simulink model "proyectolab"  (R2020a)
settings: Solver=FixedStepAuto  StartTime=0.0  StopTime=10  FixedStep=0.00001  RelTol=1e-3
values from neighbouring files (symbols this model uses):
  K = 0.0879    [dinamica.m]
undefined symbols (not defined in the file or in its folder): linsys1, Nbar
libraries: simulink x2
settings Model: Creator=USUARIO  LastModifiedBy=charlie
settings DataIOCC: ReturnWorkspaceOutputs=off
settings DebuggingCC: ArithmeticOperatorsInVariantConditions=warning
settings SFSimCC: CustomCodeUndefinedFunction=UseInterfaceOnly

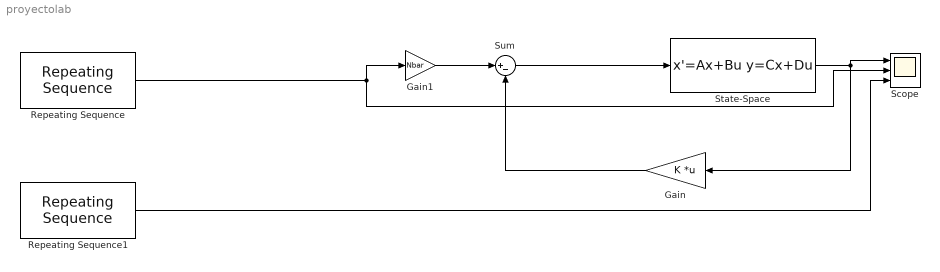
== system proyectolab ==
  Gain : Gain  Gain=K  Multiplication=Matrix(K*u) (u vector)
  Gain1 : Gain  Gain=Nbar
  Repeating Sequence : simulink/Sources/Repeating Sequence  rep_seq_t=tiempo  rep_seq_y=pos_norm
  Repeating Sequence1 : simulink/Sources/Repeating Sequence  rep_seq_t=tiempo  rep_seq_y=vel_norm
  Scope : Scope  NumInputPorts=3
  State-Space : StateSpace  A=linsys1.A  B=linsys1.B  C=eye(3)  D=[0;0;0]  InitialCondition=0
  Sum : Sum  Inputs=|+-
  wires:
  State-Space/1 -> Gain/1, Scope/1
  Gain/1 -> Sum/2
  Repeating Sequence/1 -> Gain1/1, Scope/2
  Gain1/1 -> Sum/1
  Sum/1 -> State-Space/1
  Repeating Sequence1/1 -> Scope/3
